simulink library "Lib_Cntrl_CorrectedFuelFlow_TMATS_org"  (Simulink 10.0)
settings: Solver=ode45  StartTime=0.0  StopTime=10.0  RelTol=1e-3  EnableMultiTasking=on
Description:
  | Thomas Modules
settings Model: Creator=jwchapm2  LastModifiedBy=bhisma

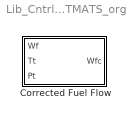
== system Lib_Cntrl_CorrectedFuelFlow_TMATS_org ==
  Corrected Fuel Flow : Subsystem  mask(T-MATS: Corrected Fuel Flow Library Block){C_TSTD_M=518.67, C_PSTD_M=14.695951}
      mask prompts: C_TSTD_M "C_TSTD_M - Standard Day Temperature [degR]"; C_PSTD_M "C_PSTD_M - Standard Day Pressure [psia]"
      mask help:
      | This block calculates corrected fuel flow.
      | Wfc = Wf /(delta*sqrt(theta))
      mask Help: web(which('Control_TMATS_CFF.html'),'-helpbrowser')

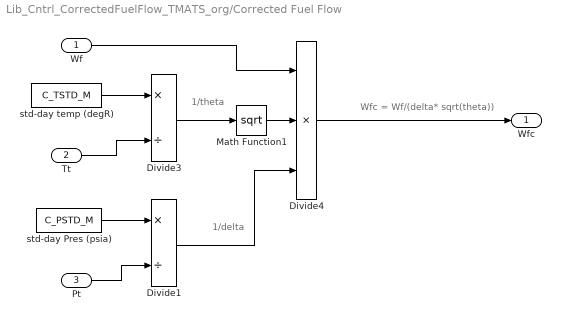
== system Lib_Cntrl_CorrectedFuelFlow_TMATS_org/Corrected Fuel Flow ==
  note: 1/delta
  note: 1/theta
  note: Wfc = Wf/(delta* sqrt(theta))
  Wf : Inport
  Tt : Inport  Port=2
  Pt : Inport  Port=3
  Divide1 : Product  Inputs=*/
  Divide3 : Product  Inputs=*/
  Divide4 : Product  Inputs=***
  Math Function1 : Math  Operator=sqrt  SaturateOnIntegerOverflow=on
  std-day Pres (psia) : Constant  Value=C_PSTD_M
  std-day temp (degR) : Constant  Value=C_TSTD_M
  Wfc : Outport
  wires:
  Pt/1 -> Divide1/2
  std-day Pres (psia)/1 -> Divide1/1
  Divide1/1 -> Divide4/3
  Divide4/1 -> Wfc/1
  Wf/1 -> Divide4/1
  Math Function1/1 -> Divide4/2
  Divide3/1 -> Math Function1/1
  std-day temp (degR)/1 -> Divide3/1
  Tt/1 -> Divide3/2
